simulink model "Sim_VSI_Resonant"  (R2025b)
settings: Solver=VariableStepAuto  StartTime=0.0  StopTime=0.3  FixedStep=Ts  RelTol=1e-3
model workspace (MAT data in the model file):
  A = [-11.6666666667  0  -333.333333333  0; 0  -11.6666666667  0  -333.333333333; 83333.3333333  0  0  0; 0  83333.3333333  0  0]
  Ard = [0.998026728428  0.0627905195293  0  0; -0.0627905195293  0.998026728428  0  0; 0  0  0.998026728428  0.0627905195293; 0  0  -0.0627905195293  0.998026728428]
  B = [333.333333333  0; 0  333.333333333; 0  0; 0  0]
  Brd = [0.000199868431248  0; -6.28111849407e-06  0; 0  0.000199868431248; 0  -6.28111849407e-06]
  C = [1  0  0  0; 0  1  0  0; 0  0  1  0; 0  0  0  1]
  Kr = [-8955.59899888  5988.13620502  -4.21296663445e-09  3.10743926347e-09; 4.74278007893e-09  -2.73306110365e-08  -8955.59899888  5988.13620502]
  Ku = [2.6094272821  4.17090298173e-13; -2.28871469679e-13  2.6094272821]
  Kx = [45.7943369878  1.07379782095e-11  1.5779453768  1.1397770542e-12; -6.12045854719e-12  45.7943369878  -9.92258509637e-13  1.5779453768]
  Ts = 0.0002
  beta_c = 3e-05
values from neighbouring files (symbols this model uses):
  Ha = [0 0 1 0 ... (first row only)    [Init_VSI_Resonant.m]
undefined symbols (not defined in the file or in its folder): P, w
libraries: simulink_extras x2
settings Model: Creator=dfigueroa  LastModifiedBy=dfigueroa

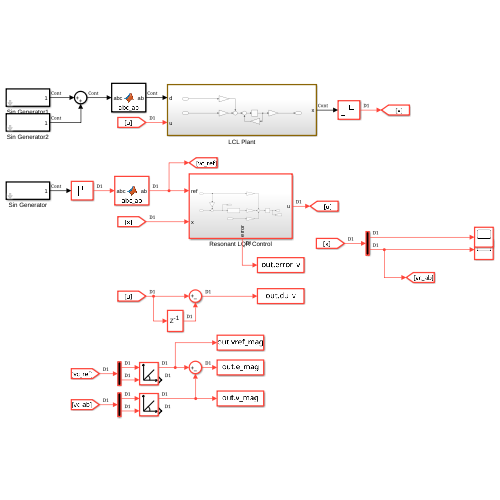
[thumbnail: Simulink's stored preview of the top-level diagram]
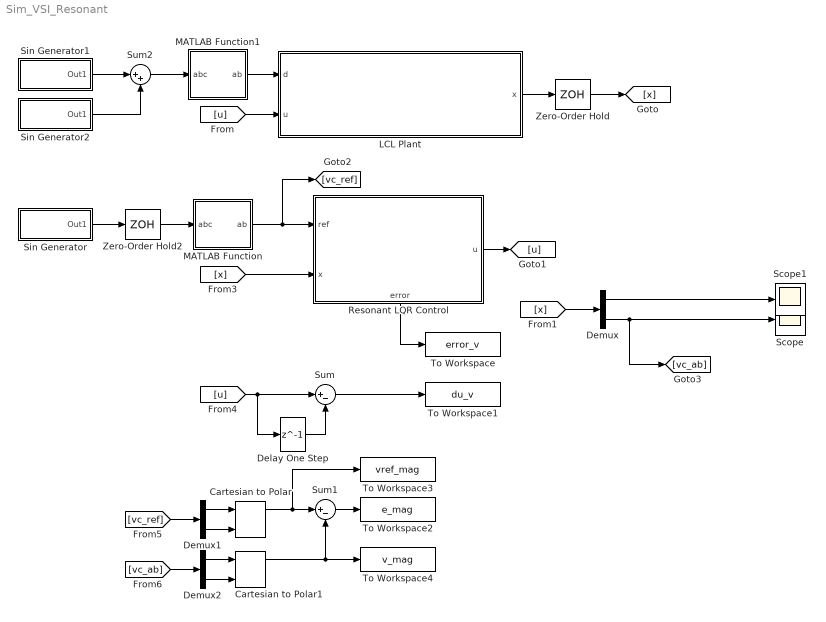
== system Sim_VSI_Resonant ==
  Cartesian to Polar : simulink_extras/Transformations/Cartesian to Polar
  Cartesian to Polar1 : simulink_extras/Transformations/Cartesian to Polar
  Delay One Step : Delay  DelayLength=1  SampleTime=Ts
  Demux : Demux  Outputs=2
  Demux1 : Demux  Outputs=2
  Demux2 : Demux  Outputs=2
  LCL Plant : Subsystem
  MATLAB Function : MATLAB Function  TreatAsAtomicUnit=on
  MATLAB Function1 : MATLAB Function  TreatAsAtomicUnit=on
  Resonant LQR Control : Subsystem
      settings: PortSchema="{\"entries\":[{\"content\":{\"sides\":[{\"content\":{\"connectorIds\":[\"In1\",\"In2\"]},\"type\":\"ConnectorPlacement.EquallySpacedRectSide\",\"uuid\":\"99a690ac-3bd0-4f81-b659-f279a9474794\"},{\"content\":{\"connectorIds\":[\"Out1\"],\"side\":\"RIGHT\"},\"type\":\"ConnectorPlacement.EquallySpacedRectSide\",\"uuid\":\"8cc57969-c53c-48c8-8db6-de6ebbedc9fa\"},{\"content\":{\"side\":\"TOP\"},\"type\":\"ConnectorPlacement.EquallySpacedRectSide\",\"uuid\":\"feb69ac5-7da0-4fd7-b564-be03e1a824d1\"},{\"content\":{\"connectorIds\":[\"Out2\"],\"side\":\"BOTTOM\"},\"type\":\"ConnectorPlacement.EquallySpacedRectSide\",\"uuid\":\"e21016e3-b19c-4730-ba77-eca85728fa6b\"}]},\"type\":\"ConnectorPlacement.EquallySpacedConnector\",\"uuid\":\"29586c0e-7c9a-4d19-baa4-f2b2392acca9\"}],\"packageUris\":[\"http://schema.mathworks.com/mf0/Connector/R2020b\"],\"version\":\"1.0\"}"
  Scope : Scope
      settings: ActiveDisplayYMinimum=-80.048593068021944  ActiveDisplayYMaximum=89.806775781162116
  Scope1 : Scope
      settings: ActiveDisplayYMinimum=-1.9729972445620159  ActiveDisplayYMaximum=2.5512495038421883
  Sin Generator : Subsystem  mask{w=w, Amp=100, Tset=0.02, Tstep=0}
      mask prompts: w "Frequency"; Amp "Reference Amplitude"; Tset "Set Time [s]"; Tstep "Step Time"
  Sin Generator1 : Subsystem  mask{w=w, Amp=0, Tset=0, Tstep=0.05}
      mask prompts: w "Frequency"; Amp "Reference Amplitude"; Tset "Set Time [s]"; Tstep "Step Time"
  Sin Generator2 : Subsystem  mask{w=3*w, Amp=0, Tset=0, Tstep=0.1}
      mask prompts: w "Frequency"; Amp "Reference Amplitude"; Tset "Set Time [s]"; Tstep "Step Time"
  Sum : Sum  Inputs=|+-
  Sum1 : Sum  Inputs=|+-
  Sum2 : Sum  Inputs=|++
  To Workspace : ToWorkspace  VariableName=error_v  SampleTime=Ts
  To Workspace1 : ToWorkspace  VariableName=du_v  SampleTime=Ts
  To Workspace2 : ToWorkspace  VariableName=e_mag  SampleTime=-1
  To Workspace3 : ToWorkspace  VariableName=vref_mag  SampleTime=Ts
  To Workspace4 : ToWorkspace  VariableName=v_mag  SampleTime=Ts
  Zero-Order Hold : ZeroOrderHold  SampleTime=Ts
  Zero-Order Hold2 : ZeroOrderHold  SampleTime=Ts
  wires:
  Demux/2 -> [vc_ab], Scope/1
  [x] -> Demux/1
  Zero-Order Hold/1 -> [x]
  Zero-Order Hold2/1 -> MATLAB Function/1(abc)
  LCL Plant/1(x) -> Zero-Order Hold/1
  [u] -> LCL Plant/2(u)
  [x] -> Resonant LQR Control/2(x)
  Resonant LQR Control/1(u) -> [u]
  Sin Generator/1(Out1) -> Zero-Order Hold2/1
  MATLAB Function/1(ab) -> [vc_ref], Resonant LQR Control/1(ref)
  [u] -> Delay One Step/1, Sum/1
  Delay One Step/1 -> Sum/2
  Resonant LQR Control/2(error) -> To Workspace/1
  [vc_ref] -> Demux1/1
  Demux1/1 -> Cartesian to Polar/1
  Demux1/2 -> Cartesian to Polar/2
  Cartesian to Polar/1 -> To Workspace3/1, Sum1/1
  Sum1/1 -> To Workspace2/1
  Demux2/1 -> Cartesian to Polar1/1
  [vc_ab] -> Demux2/1
  Demux2/2 -> Cartesian to Polar1/2
  Cartesian to Polar1/1 -> Sum1/2, To Workspace4/1
  Sin Generator1/1(Out1) -> Sum2/1
  Sum/1 -> To Workspace1/1
  MATLAB Function1/1(ab) -> LCL Plant/1(d)
  Sin Generator2/1(Out1) -> Sum2/2
  Sum2/1 -> MATLAB Function1/1(abc)
  Demux/1 -> Scope1/1

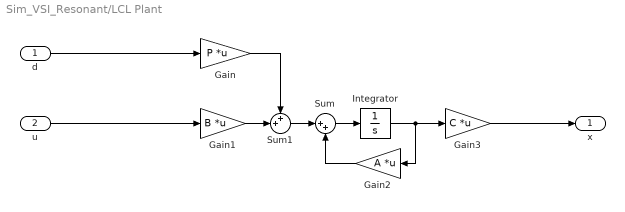
== system Sim_VSI_Resonant/LCL Plant ==
  d : Inport
  u : Inport  Port=2
  Gain : Gain  Gain=P  Multiplication=Matrix(K*u)
  Gain1 : Gain  Gain=B  Multiplication=Matrix(K*u)
  Gain2 : Gain  Gain=A  Multiplication=Matrix(K*u)
  Gain3 : Gain  Gain=C  Multiplication=Matrix(K*u)
  Integrator : Integrator
  Sum : Sum  Inputs=|++
  Sum1 : Sum  Inputs=++|
  x : Outport
  wires:
  u/1 -> Gain1/1
  Gain2/1 -> Sum/2
  Gain/1 -> Sum1/1
  Sum/1 -> Integrator/1
  Integrator/1 -> Gain3/1, Gain2/1
  d/1 -> Gain/1
  Sum1/1 -> Sum/1
  Gain1/1 -> Sum1/2
  Gain3/1 -> x/1

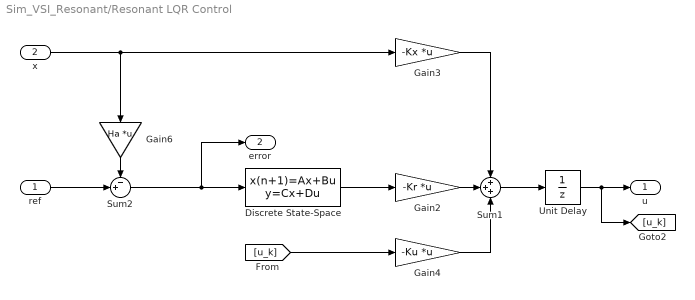
== system Sim_VSI_Resonant/Resonant LQR Control ==
  ref : Inport
  x : Inport  Port=2
  Discrete State-Space : DiscreteStateSpace  A=Ard  B=Brd  C=eye(4)  D=zeros(4,2)  SampleTime=Ts
  Gain2 : Gain  Gain=-Kr  Multiplication=Matrix(K*u)
  Gain3 : Gain  Gain=-Kx  Multiplication=Matrix(K*u)
  Gain4 : Gain  Gain=-Ku  Multiplication=Matrix(K*u)
  Gain6 : Gain  Gain=Ha  Multiplication=Matrix(K*u)
  Sum1 : Sum  Inputs=+++
  Sum2 : Sum  Inputs=-+|
  Unit Delay : UnitDelay  SampleTime=Ts  HasFrameUpgradeWarning=on
  u : Outport
  error : Outport  Port=2
  wires:
  x/1 -> Gain6/1, Gain3/1
  Gain6/1 -> Sum2/1
  Unit Delay/1 -> [u_k], u/1
  ref/1 -> Sum2/2
  Gain2/1 -> Sum1/2
  Gain3/1 -> Sum1/1
  Gain4/1 -> Sum1/3
  [u_k] -> Gain4/1
  Sum1/1 -> Unit Delay/1
  Sum2/1 -> error/1, Discrete State-Space/1
  Discrete State-Space/1 -> Gain2/1

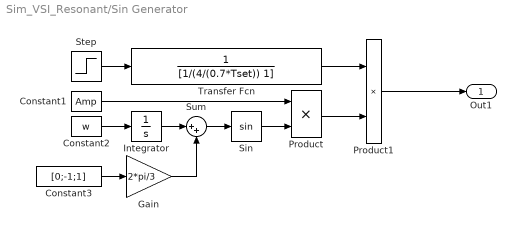
== system Sim_VSI_Resonant/Sin Generator ==
  Constant1 : Constant  Value=Amp
  Constant2 : Constant  Value=w
  Constant3 : Constant  Value=[0;-1;1]
  Gain : Gain  Gain=2*pi/3
  Integrator : Integrator
  Product : Product
  Product1 : Product
  Sin : Trigonometry
  Step : Step  Time=Tstep  SampleTime=0
  Sum : Sum  Inputs=|++
  Transfer Fcn : TransferFcn  Denominator=[1/(4/(0.7*Tset)) 1]
  Out1 : Outport
  wires:
  Sum/1 -> Sin/1
  Transfer Fcn/1 -> Product1/1
  Constant2/1 -> Integrator/1
  Integrator/1 -> Sum/1
  Constant1/1 -> Product/1
  Constant3/1 -> Gain/1
  Product1/1 -> Out1/1
  Gain/1 -> Sum/2
  Step/1 -> Transfer Fcn/1
  Sin/1 -> Product/2
  Product/1 -> Product1/2

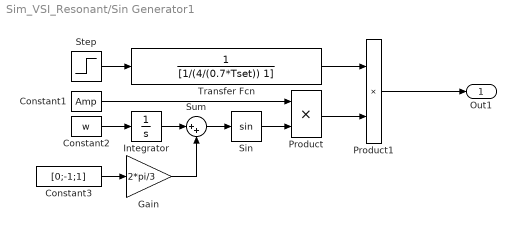
== system Sim_VSI_Resonant/Sin Generator1 ==
  Constant1 : Constant  Value=Amp
  Constant2 : Constant  Value=w
  Constant3 : Constant  Value=[0;-1;1]
  Gain : Gain  Gain=2*pi/3
  Integrator : Integrator
  Product : Product
  Product1 : Product
  Sin : Trigonometry
  Step : Step  Time=Tstep  SampleTime=0
  Sum : Sum  Inputs=|++
  Transfer Fcn : TransferFcn  Denominator=[1/(4/(0.7*Tset)) 1]
  Out1 : Outport
  wires:
  Product/1 -> Product1/2
  Sin/1 -> Product/2
  Step/1 -> Transfer Fcn/1
  Gain/1 -> Sum/2
  Product1/1 -> Out1/1
  Constant3/1 -> Gain/1
  Constant1/1 -> Product/1
  Integrator/1 -> Sum/1
  Constant2/1 -> Integrator/1
  Transfer Fcn/1 -> Product1/1
  Sum/1 -> Sin/1

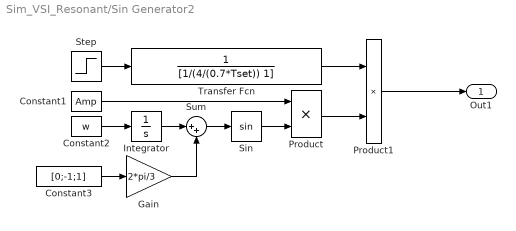
== system Sim_VSI_Resonant/Sin Generator2 ==
  Constant1 : Constant  Value=Amp
  Constant2 : Constant  Value=w
  Constant3 : Constant  Value=[0;-1;1]
  Gain : Gain  Gain=2*pi/3
  Integrator : Integrator
  Product : Product
  Product1 : Product
  Sin : Trigonometry
  Step : Step  Time=Tstep  SampleTime=0
  Sum : Sum  Inputs=|++
  Transfer Fcn : TransferFcn  Denominator=[1/(4/(0.7*Tset)) 1]
  Out1 : Outport
  wires:
  Sum/1 -> Sin/1
  Transfer Fcn/1 -> Product1/1
  Constant2/1 -> Integrator/1
  Integrator/1 -> Sum/1
  Constant1/1 -> Product/1
  Constant3/1 -> Gain/1
  Product1/1 -> Out1/1
  Gain/1 -> Sum/2
  Step/1 -> Transfer Fcn/1
  Sin/1 -> Product/2
  Product/1 -> Product1/2

== matlab function Sim_VSI_Resonant/MATLAB Function ==
  data: abc input; ab output
function ab = abc_ab(abc)
    alpha = (2*abc(1) - abc(2) - abc(3))/3;
    beta = (abc(2) - abc(3))/sqrt(3);
ab = [alpha;beta];

== matlab function Sim_VSI_Resonant/MATLAB Function1 ==
  data: abc input; ab output
function ab = abc_ab(abc)
    alpha = (2*abc(1) - abc(2) - abc(3))/3;
    beta = (abc(2) - abc(3))/sqrt(3);
ab = [alpha;beta];
